simulink model "joint_control_sl"  (R2015a)
settings: Solver=ode45  StartTime=0.0  StopTime=1.0  RelTol=1e-3
values from neighbouring files (symbols this model uses):
  T = T * subs(T_gen, {'alph' 'theta'  'd'  'a'},{ alpha_i(cnt) theta_i(cnt) d_i(cnt)  a_i(cnt)})    [FK.m]    (also in getTF.m = [R_12 tr_12; 0 0 0 1]; interpolate.m = max(abs(Q(:,3)-Q(:,1))); kinematika.m = FK(as, ds, thetas, alphas); test_closest_q.m = Mask*T_)
settings Model: Creator=marki  LastModifiedBy=marki

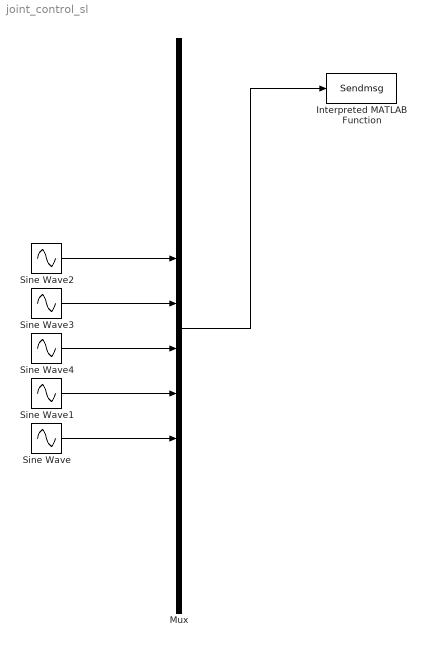
== system joint_control_sl ==
  Interpreted MATLAB Function : MATLABFcn  MATLABFcn=Sendmsg  OutputDimensions=0
  Mux : Mux  Inputs=12
  Sine Wave : Sin  Amplitude=0.1  SampleTime=T
  Sine Wave1 : Sin  Amplitude=0  Phase=pi/2  SampleTime=T  VectorParams1D=off
  Sine Wave2 : Sin  Phase=pi  SampleTime=T
  Sine Wave3 : Sin  Phase=3*pi/2  SampleTime=T
  Sine Wave4 : Sin  Phase=3*pi/2  SampleTime=T
  wires:
  Mux/1 -> Interpreted MATLAB Function/1
  Sine Wave3/1 -> Mux/6
  Sine Wave4/1 -> Mux/7
  Sine Wave2/1 -> Mux/5
  Sine Wave1/1 -> Mux/8
  Sine Wave/1 -> Mux/9
